simulink model "FlybackBoost"  (R2023b)
settings: Solver=VariableStepAuto  StartTime=0.0  StopTime=0.1  RelTol=1e-3
libraries: spsSeriesRLCBranchLib x8, spsDiodeLib x3, spsMosfetLib x2, eePwmGenerator x2, spsVariableRatioTransformerLib x2, spsVoltageMeasurementLib x2, spsControlledVoltageSourceLib x1, sps_lib x1
settings Model: SimulationMode=accelerator  Creator=32295  LastModifiedBy=32295
settings SolverCC: ZeroCrossAlgorithm=Adaptive
settings DebuggingCC: IgnoredZcDiagnostic=none

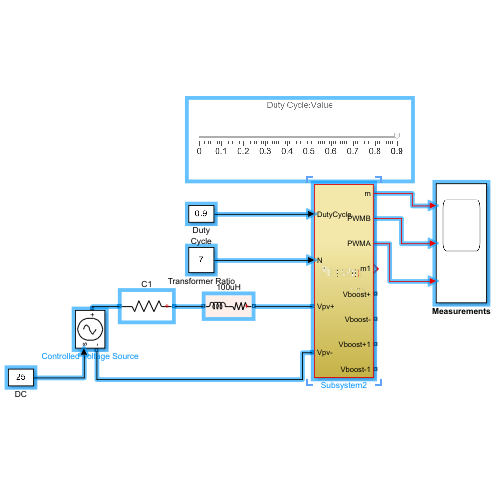
[thumbnail: Simulink's stored preview of the top-level diagram]
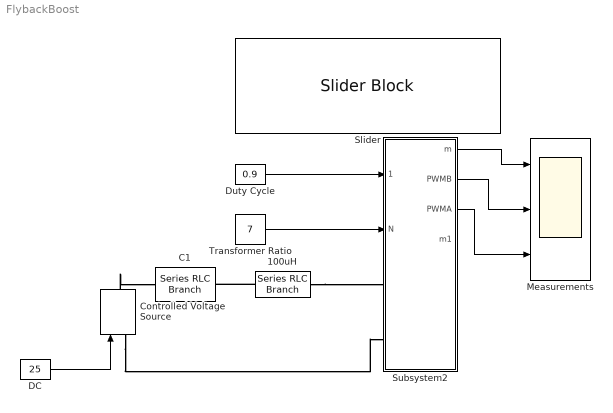
== system FlybackBoost ==
  100uH : spsSeriesRLCBranchLib/Series RLC Branch  LConnTagsString=__new0  RConnTagsString=__new0  BranchType=RL  Resistance=0.05  Inductance=100e-6  SetiL0=off  InitialCurrent=0  Capacitance=1e-6  Setx0=off  InitialVoltage=0  Measurements=None
  C1 : spsSeriesRLCBranchLib/Series RLC Branch  LConnTagsString=__new0  RConnTagsString=__new0  BranchType=R  Resistance=1e-6  Inductance=1e-3  SetiL0=off  InitialCurrent=0  Capacitance=680e-6  Setx0=off  InitialVoltage=20  Measurements=None
  Controlled Voltage Source : spsControlledVoltageSourceLib/Controlled Voltage Source  Initialize=on  Source_Type=DC  Amplitude=25  Phase=0  Frequency=0  Measurements=None
  DC : Constant  Value=25
  Duty Cycle : Constant  Value=0.9
  Measurements : Scope  NumInputPorts=3
  Slider : SliderBlock  ScaleMax=0.9  TickInterval=0.10000000000000001
  Subsystem2 : Subsystem
  Transformer Ratio : Constant  Value=7
  wires:
  DC/1 -> Controlled Voltage Source/1
  Duty Cycle/1 -> Subsystem2/1(DutyCycle)
  Transformer Ratio/1 -> Subsystem2/2(N)
  Subsystem2/1(m) -> Measurements/1
  Subsystem2/2(PWMB) -> Measurements/2
  Subsystem2/3(PWMA) -> Measurements/3
  connections:
  Controlled Voltage Source/LConn1 -- Subsystem2/LConn2
  Controlled Voltage Source/RConn1 -- C1/RConn1
  100uH/RConn1 -- C1/LConn1
  100uH/LConn1 -- Subsystem2/LConn1

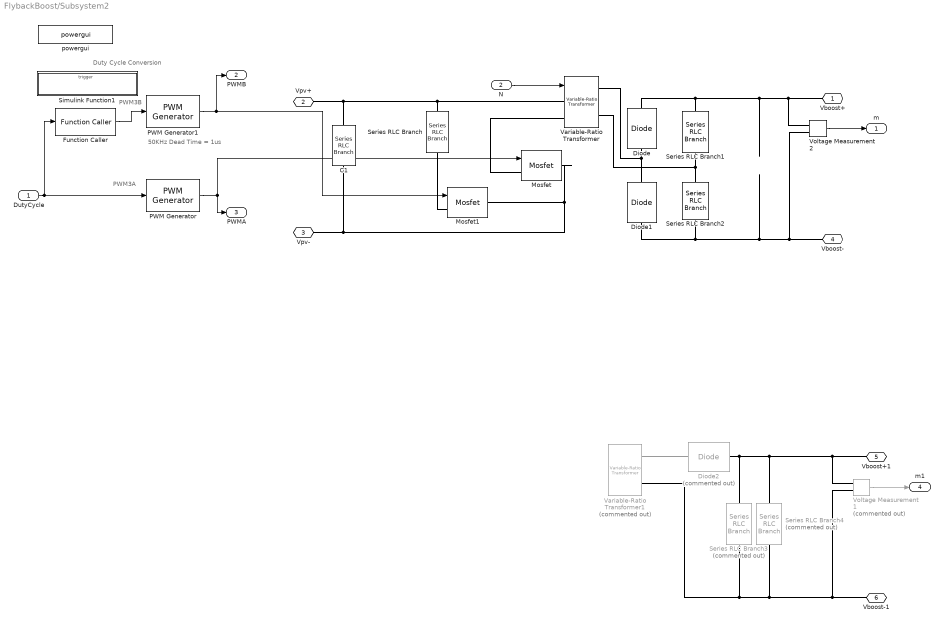
== system FlybackBoost/Subsystem2 ==
  note: Duty Cycle Conversion
  note: 50KHz
      | Dead Time = 1us
  note: PWM3B
  note: PWM3A
  DutyCycle : Inport
  N : Inport  Port=2
  C1 : spsSeriesRLCBranchLib/Series RLC Branch  LConnTagsString=__new0  RConnTagsString=__new0  BranchType=C  Resistance=1e-3  Inductance=1e-3  SetiL0=off  InitialCurrent=0  Capacitance=10e-6  Setx0=off  InitialVoltage=20  Measurements=None
  Diode : spsDiodeLib/Diode  Ron=0.001  Lon=0  Vf=0.6  IC=0  UseSnubber=0  Rs=500  Cs=250e-9  Measurements=off
  Diode1 : spsDiodeLib/Diode  Ron=0.001  Lon=0  Vf=0.6  IC=0  UseSnubber=0  Rs=500  Cs=250e-9  Measurements=off
  Diode2 : spsDiodeLib/Diode  Commented=on  Ron=0.001  Lon=0  Vf=0.6  IC=0  UseSnubber=0  Rs=500  Cs=250e-9  Measurements=off
  Function Caller : FunctionCaller  FunctionPrototype=y = DutyConv(x)  InputArgumentSpecifications=<Enter example>  OutputArgumentSpecifications=<Enter example>
  Mosfet : spsMosfetLib/Mosfet  Ron=0.1  Lon=0  Rd=0.01  Vfd=0  IC=0  Rs=1e5  Cs=inf  Measurements=off
  Mosfet1 : spsMosfetLib/Mosfet  Ron=0.1  Lon=0  Rd=0.01  Vfd=0  IC=0  Rs=1e5  Cs=inf  Measurements=off
  PWM Generator : eePwmGenerator/PWM Generator  CarrCount=Up  Tper=20e-6  Tdelay=10e-6  Ts=1e-10
  PWM Generator1 : eePwmGenerator/PWM Generator  CarrCount=Up  Tper=20e-6  Tdelay=9e-6  Ts=1e-10
  Series RLC Branch : spsSeriesRLCBranchLib/Series RLC Branch  LConnTagsString=__new0  RConnTagsString=__new0  BranchType=C  Resistance=1  Inductance=1e-3  SetiL0=off  InitialCurrent=0  Capacitance=1e-6  Setx0=off  InitialVoltage=0  Measurements=None
  Series RLC Branch1 : spsSeriesRLCBranchLib/Series RLC Branch  LConnTagsString=__new0  RConnTagsString=__new0  BranchType=C  Resistance=1  Inductance=1e-3  SetiL0=off  InitialCurrent=0  Capacitance=3e-6  Setx0=off  InitialVoltage=0  Measurements=None
  Series RLC Branch2 : spsSeriesRLCBranchLib/Series RLC Branch  LConnTagsString=__new0  RConnTagsString=__new0  BranchType=C  Resistance=1  Inductance=1e-3  SetiL0=off  InitialCurrent=0  Capacitance=3e-6  Setx0=off  InitialVoltage=0  Measurements=None
  Series RLC Branch3 : spsSeriesRLCBranchLib/Series RLC Branch  Commented=on  LConnTagsString=__new0  RConnTagsString=__new0  BranchType=C  Resistance=1  Inductance=1e-3  SetiL0=off  InitialCurrent=0  Capacitance=1640e-6  Setx0=off  InitialVoltage=0  Measurements=None
  Series RLC Branch4 : spsSeriesRLCBranchLib/Series RLC Branch  Commented=on  LConnTagsString=__new0  RConnTagsString=__new0  BranchType=R  Resistance=10  Inductance=1e-3  SetiL0=off  InitialCurrent=0  Capacitance=10e-6  Setx0=off  InitialVoltage=0  Measurements=None
  Simulink Function1 : Subsystem  TreatAsAtomicUnit=on
  Variable-Ratio Transformer : spsVariableRatioTransformerLib/Variable-Ratio Transformer
      settings: LibrarySourceBlock=|
      | sps_lib/Passives/Variable-Ratio
      | Transformer
  Variable-Ratio Transformer1 : spsVariableRatioTransformerLib/Variable-Ratio Transformer  Commented=on
      settings: LibrarySourceBlock=|
      | sps_lib/Passives/Variable-Ratio
      | Transformer
  Voltage Measurement1 : spsVoltageMeasurementLib/Voltage Measurement  Commented=on  PhasorSimulation=off  OutputType=Complex  PSBequivalent=0
  Voltage Measurement2 : spsVoltageMeasurementLib/Voltage Measurement  PhasorSimulation=off  OutputType=Complex  PSBequivalent=0
  powergui : sps_lib/powergui  Priority=1  SimulationMode=Discrete  SampleTime=1e-5  frequency=60  Iterations=50  frequencyindice=0  Pbase=100e6  ErrMax=1e-4  UnitsV=kV  UnitsW=MW  buscounter=0  FunctionMessages=off  echomessages=off  EnableUseOfTLC=off  CurrentSourceSwitches=off  DisableSnubberDevices=off  DisableRonSwitches=off  DisableVfSwitches=off  DisplayEquations=off  AutomaticDiscreteSolvers=off  SolverType=Tustin  Interpol=off  ExternalGateDelay=off  methode=off  Ts=0  x0status=blocks  SPID=off  SwTol=0  HookPort=off  NonlinearTolerance=1e-4  nMaxIteration=100  ContinueOnMaxIteration=off  RestoreLinks=warning  ResistiveCurrentMeasurement=off  Frange=[0:2:500]  Ylog=off  Xlog=on  ShowGrid=off  save=off  variable=ZData  structure=0  ZoomFFT=on  StartTime=0.0  cycles=1  DisplayStyle=1  fundamental=60  FreqAxis=off  MaxFrequency=1000  frequencyindicesteady=1  RmsSteady=1  display=off
  Vboost+ : PMIOPort  Side=Right
  Vpv+ : PMIOPort  Port=2  Side=Left
  Vpv- : PMIOPort  Port=3  Side=Left
  Vboost- : PMIOPort  Port=4  Side=Right
  Vboost+1 : PMIOPort  Port=5  Side=Right
  Vboost-1 : PMIOPort  Port=6  Side=Right
  m : Outport  VectorParamsAs1DForOutWhenUnconnected=off
  PWMB : Outport  Port=2  VectorParamsAs1DForOutWhenUnconnected=off
  PWMA : Outport  Port=3  VectorParamsAs1DForOutWhenUnconnected=off
  m1 : Outport  Port=4  VectorParamsAs1DForOutWhenUnconnected=off
  wires:
  N/1 -> Variable-Ratio Transformer/1
  DutyCycle/1 -> Function Caller/1, PWM Generator/1
  Voltage Measurement2/1 -> m/1
  PWM Generator/1 -> Mosfet/1, PWMA/1
  PWM Generator1/1 -> Mosfet1/1, PWMB/1
  Function Caller/1 -> PWM Generator1/1
  Voltage Measurement1/1 -> m1/1
  connections:
  Series RLC Branch1/RConn1 -- Series RLC Branch2/LConn1 -- Variable-Ratio Transformer/RConn2
  Diode/LConn1 -- Diode1/RConn1 -- Variable-Ratio Transformer/RConn1
  Mosfet/RConn1 -- Vpv-/RConn1 -- C1/RConn1 -- Mosfet1/RConn1
  Diode1/LConn1 -- Voltage Measurement2/LConn2 -- Vboost-/RConn1 -- Series RLC Branch2/RConn1
  Series RLC Branch1/LConn1 -- Voltage Measurement2/LConn1 -- Vboost+/RConn1 -- Diode/RConn1
  C1/LConn1 -- Variable-Ratio Transformer/LConn1 -- Series RLC Branch/LConn1 -- Vpv+/RConn1
  Mosfet/LConn1 -- Variable-Ratio Transformer/LConn2
  Mosfet1/LConn1 -- Series RLC Branch/RConn1
  Vboost-1/RConn1 -- Voltage Measurement1/LConn2 -- Series RLC Branch4/RConn1 -- Series RLC Branch3/RConn1 -- Variable-Ratio Transformer1/RConn2
  Diode2/RConn1 -- Series RLC Branch3/LConn1 -- Voltage Measurement1/LConn1 -- Vboost+1/RConn1 -- Series RLC Branch4/LConn1
  Diode2/LConn1 -- Variable-Ratio Transformer1/RConn1

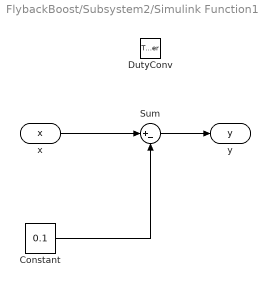
== system FlybackBoost/Subsystem2/Simulink Function1 ==
  DutyConv : TriggerPort  TriggerType=function-call  IsSimulinkFunction=on  FunctionName=DutyConv  FunctionVisibility=scoped  VariantControl=(inherit)
  Constant : Constant  Value=0.1
  Sum : Sum  Inputs=|+-
  x : ArgIn  DisableCoverage=on  ArgumentName=x
  y : ArgOut  DisableCoverage=on  ArgumentName=y
  wires:
  Constant/1 -> Sum/2
  x/1 -> Sum/1
  Sum/1 -> y/1
